simulink model "blockdiagram"  (R2020a)
settings: Solver=ode4  StartTime=0.0  StopTime=12  FixedStep=0.001  RelTol=1e-3
values from neighbouring files (symbols this model uses):
  B = 0.05    [ProblemA.m]
  J = 0.1    [ProblemA.m]
  L2 = (Lmax-Lmin)/2    (= 0.04)    [ProblemA.m]
  theta_m0 = 0    [ProblemA.m]
undefined symbols (not defined in the file or in its folder): sigbuilder_block
libraries: simulink x6
(part 1 of 2)
settings Model: Creator=IM SEYEONG  LastModifiedBy=IM SEYEONG

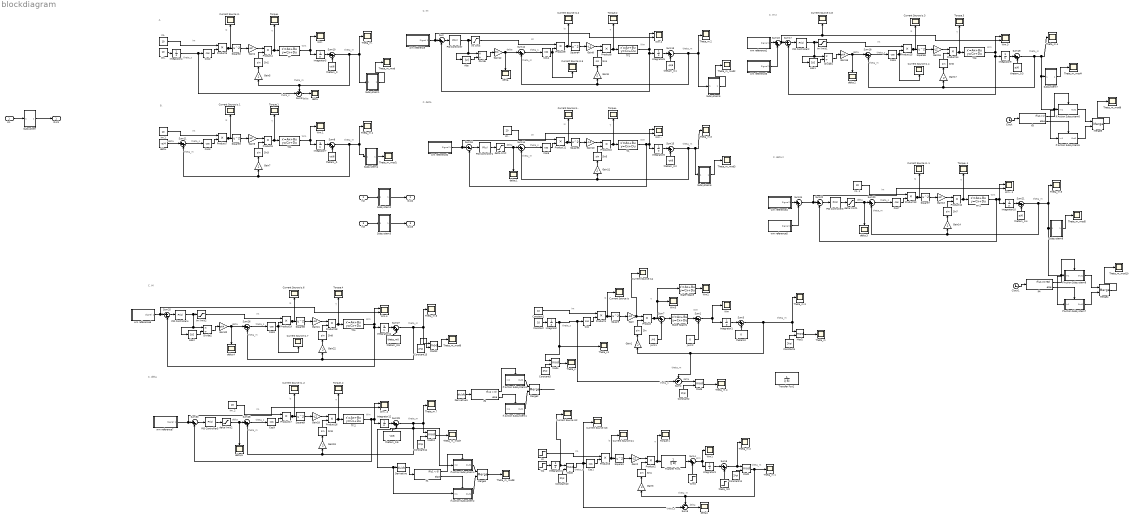
== system blockdiagram ==
  note: Wm
  note: T
  note: theta_m
  note: is
  note: theta_s
  note: Im
  note: theta_m
  note: theta_m
  note: Wm
  note: is
  note: theta_s
  note: delta
  note: T
  note: Im
  note: theta_s
  note: theta_m
  note: delta
  note: theta_s
  note: Wm
  note: theta_m
  note: theta_m
  note: is
  note: theta_s
  note: theta_s
  note: delta
  note: T
  note: Im
  note: A.
  note: B.
  note: T
  note: Im
  note: theta_m
  note: theta_s
  note: theta_m
  note: is
  note: Wm
  note: delta
  note: T
  note: theta_s
  note: theta_m
  note: Im
  note: C. IM
  note: is
  note: Wm
  note: delta
  note: theta_m
  note: T
  note: theta_s
  note: theta_m
  note: Im
  note: C. delta
  note: is
  note: Wm
  note: delta
  note: theta_m
  note: T
  note: C. delta 2
  note: delta
  note: Im
  note: theta_s
  note: theta_m
  note: theta_m
  note: Im
  note: C. IM 2
  note: is
  note: Wm
  note: Wm
  note: is
  note: T
  note: theta_s
  note: theta_m
  note: theta_m
  note: delta
  note: T
  note: C. delta
  note: delta
  note: Im
  note: theta_s
  note: theta_m
  note: theta_m
  note: Im
  note: C. IM
  note: is
  note: Wm
  note: Wm
  note: is
  note: T
  note: theta_s
  note: theta_m
  note: theta_m
  note: delta
  In1 : Inport
  In2 : Inport  Port=2
  In3 : Inport  Port=3
  Abs : Abs
  Abs1 : Abs
  Abs2 : Abs
  Clock : Clock
  Clock1 : Clock
  Constant : Constant  Value=10
  Constant1 : Constant  Value=10
  Constant{2,4..5,10..11,13..14} (7 alike) : Constant  Value=2*pi
  Cos{,1..9} (10 alike) : Trigonometry  Operator=cos
  Current Source is{,1..4} (5 alike) : Scope
  Current Source is.{,1..8} (9 alike) : Scope
  Current Source is.. : Scope
  Current Source is..1 : Scope
  Current Source is..2 : Scope
  Derivative : Derivative
  Derivative1 : Derivative
  Divide : Product  Inputs=*/
  Divide1 : Product  Inputs=*/
  Divide2 : Product  Inputs=*/
  Gain{,2,4,6,8,10,13,16,18,21} (10 alike) : Gain  Gain=-L2
  Gain{1,3,5,7,9,11,14,17,19,22} (10 alike) : Gain  Gain=2
  Gain12 : Gain  Gain=pi/4
  Gain15 : Gain  Gain=pi/4
  Gain20 : Gain  Gain=pi/4
  If Action Subsystem1 : Subsystem  TreatAsAtomicUnit=on
  If Action Subsystem2 : Subsystem  TreatAsAtomicUnit=on
  If Action Subsystem3 : Subsystem  TreatAsAtomicUnit=on
  If Action Subsystem4 : Subsystem  TreatAsAtomicUnit=on
  If Action Subsystem5 : Subsystem  TreatAsAtomicUnit=on
  If Action Subsystem6 : Subsystem  TreatAsAtomicUnit=on
  If Action Subsystem7 : Subsystem  TreatAsAtomicUnit=on
  If Action Subsystem8 : Subsystem  TreatAsAtomicUnit=on
  If1 : If  IfExpression=u1 < 0
  If2 : If  IfExpression=u1 < 0
  If3 : If  IfExpression=u1<1
  If4 : If  IfExpression=u1<0.732
  Im : Step  Time=0  After=10  SampleTime=0
  Im limit : Saturate  UpperLimit=20  LowerLimit=-20
  Im limit1 : Saturate  UpperLimit=20  LowerLimit=-20
  Im limit2 : Saturate  UpperLimit=20  LowerLimit=-20
  Im. : Constant  Value=10
  Im.. : Constant  Value=20
  Im..1 : Constant  Value=20
  Im..2 : Constant  Value=20
  Im.1 : Constant  Value=10
  Integrator{,1..12} (13 alike) : Integrator
  Jwm1 : Constant  Value=J*0
  Jwm2 : Constant  Value=0
  Merge{1..4} (4 alike) : Merge
  Mod{1..2,4..5,12..13} (6 alike) : Math  Operator=mod  SaturateOnIntegerOverflow=on
  Mod3 : Math  Operator=mod  OutputSignalType=real  SaturateOnIntegerOverflow=on
  PID Controller : simulink/Continuous/PID Controller  Controller=PI  Form=Parallel  TimeDomain=Continuous-time  UseExternalTs=off  SampleTime=-1  IntegratorMethod=Forward Euler  FilterMethod=Forward Euler  ControllerParametersSource=internal  P=4  I=0.9  D=0  UseFilter=on  N=100  TunerSelectOption=Transfer Function Based (PID Tuner App)  InitialConditionSource=internal  InitialConditionForIntegrator=0  InitialConditionForFilter=0  DifferentiatorICPrevScaledInput=0  ExternalReset=none  TrackingMode=off  Kt=1  LimitOutput=off  UpperSaturationLimit=inf  LowerSaturationLimit=-inf  LinearizeAsGain=on  AntiWindupMode=none  Kb=1  POutMin=[]  POutMax=[]  IOutMin=[]  IOutMax=[]  DOutMin=[]  DOutMax=[]  NOutMin=[]  NOutMax=[]  SumOutMin=[]  SumOutMax=[]  SaturationOutMin=[]  SaturationOutMax=[]  PParamMin=[]  PParamMax=[]  IParamMin=[]  IParamMax=[]  DParamMin=[]  DParamMax=[]  NParamMin=[]  NParamMax=[]  KbParamMin=[]  KbParamMax=[]  KtParamMin=[]  KtParamMax=[]  KbOutMin=[]  KbOutMax=[]  KtOutMin=[]  KtOutMax=[]  IntegratorOutMin=[]  IntegratorOutMax=[]  FilterOutMin=[]  FilterOutMax=[]  SumI1OutMin=[]  SumI1OutMax=[]  SumI2OutMin=[]  SumI2OutMax=[]  SumI3OutMin=[]  SumI3OutMax=[]  SumI4OutMin=[]  SumI4OutMax=[]  SumDOutMin=[]  SumDOutMax=[]  DifferentiatorOutMin=[]  DifferentiatorOutMax=[]  FilterDiffOutCoefMin=[]  FilterDiffOutCoefMax=[]  ReciprocalOutMin=[]  ReciprocalOutMax=[]  SumDenOutMin=[]  SumDenOutMax=[]  SumNumOutMin=[]  SumNumOutMax=[]  DivideOutMin=[]  DivideOutMax=[]  UdiffTsProdOutMin=[]  UdiffTsProdOutMax=[]  NTsProdOutMin=[]  NTsProdOutMax=[]  UintegralTsProdOutMin=[]  UintegralTsProdOutMax=[]  UngainTsProdOutMin=[]  UngainTsProdOutMax=[]  IntegratorContinuousStateAttributes=''  IntegratorStateMustResolveToSignalObject=off  IntegratorRTWStateStorageClass=Auto  FilterContinuousStateAttributes=''  FilterStateMustResolveToSignalObject=off  FilterRTWStateStorageClass=Auto  ParallelPVariant=InternalParameters  IdealPVariant=Disabled  IVariant=InternalParameters  DVariant=Disabled  IntegratorVariant=Continuous  SatVariant=Disabled  AWVariant=Passthrough  PCopyVariant=Disabled  TRVariant=Disabled  FdbkBlocksVariant=Forward  IdealPFdbkVariant=Disabled  SatFdbkVariant=Disabled  DerivativeFilterVariant=Disabled  NVariant=Disabled  NCopyVariant=Disabled_SignalSpec  FilterICVariant=Disabled  IntegratorICVariant=InternalICs  ExternalResetVariant=Disabled  TRSumVariant=Passthrough  SumFdbkVariant=Disabled  SumVariant=Sum_PI  TsampFilterVariant=InternalTs  TsampNgainVariant=Passthrough  TsampIntegralVariant=Passthrough
  PID Controller1 : simulink/Continuous/PID Controller  Controller=PI  Form=Parallel  TimeDomain=Continuous-time  UseExternalTs=off  SampleTime=-1  IntegratorMethod=Forward Euler  FilterMethod=Forward Euler  ControllerParametersSource=internal  P=1  I=0.05  D=0  UseFilter=on  N=100  TunerSelectOption=Transfer Function Based (PID Tuner App)  InitialConditionSource=internal  InitialConditionForIntegrator=0  InitialConditionForFilter=0  DifferentiatorICPrevScaledInput=0  ExternalReset=none  TrackingMode=off  Kt=1  LimitOutput=off  UpperSaturationLimit=inf  LowerSaturationLimit=-inf  LinearizeAsGain=on  AntiWindupMode=none  Kb=1  POutMin=[]  POutMax=[]  IOutMin=[]  IOutMax=[]  DOutMin=[]  DOutMax=[]  NOutMin=[]  NOutMax=[]  SumOutMin=[]  SumOutMax=[]  SaturationOutMin=[]  SaturationOutMax=[]  PParamMin=[]  PParamMax=[]  IParamMin=[]  IParamMax=[]  DParamMin=[]  DParamMax=[]  NParamMin=[]  NParamMax=[]  KbParamMin=[]  KbParamMax=[]  KtParamMin=[]  KtParamMax=[]  KbOutMin=[]  KbOutMax=[]  KtOutMin=[]  KtOutMax=[]  IntegratorOutMin=[]  IntegratorOutMax=[]  FilterOutMin=[]  FilterOutMax=[]  SumI1OutMin=[]  SumI1OutMax=[]  SumI2OutMin=[]  SumI2OutMax=[]  SumI3OutMin=[]  SumI3OutMax=[]  SumI4OutMin=[]  SumI4OutMax=[]  SumDOutMin=[]  SumDOutMax=[]  DifferentiatorOutMin=[]  DifferentiatorOutMax=[]  FilterDiffOutCoefMin=[]  FilterDiffOutCoefMax=[]  ReciprocalOutMin=[]  ReciprocalOutMax=[]  SumDenOutMin=[]  SumDenOutMax=[]  SumNumOutMin=[]  SumNumOutMax=[]  DivideOutMin=[]  DivideOutMax=[]  UdiffTsProdOutMin=[]  UdiffTsProdOutMax=[]  NTsProdOutMin=[]  NTsProdOutMax=[]  UintegralTsProdOutMin=[]  UintegralTsProdOutMax=[]  UngainTsProdOutMin=[]  UngainTsProdOutMax=[]  IntegratorContinuousStateAttributes=''  IntegratorStateMustResolveToSignalObject=off  IntegratorRTWStateStorageClass=Auto  FilterContinuousStateAttributes=''  FilterStateMustResolveToSignalObject=off  FilterRTWStateStorageClass=Auto  ParallelPVariant=InternalParameters  IdealPVariant=Disabled  IVariant=InternalParameters  DVariant=Disabled  IntegratorVariant=Continuous  SatVariant=Disabled  AWVariant=Passthrough  PCopyVariant=Disabled  TRVariant=Disabled  FdbkBlocksVariant=Forward  IdealPFdbkVariant=Disabled  SatFdbkVariant=Disabled  DerivativeFilterVariant=Disabled  NVariant=Disabled  NCopyVariant=Disabled_SignalSpec  FilterICVariant=Disabled  IntegratorICVariant=InternalICs  ExternalResetVariant=Disabled  TRSumVariant=Passthrough  SumFdbkVariant=Disabled  SumVariant=Sum_PI  TsampFilterVariant=InternalTs  TsampNgainVariant=Passthrough  TsampIntegralVariant=Passthrough
  PID Controller2 : simulink/Continuous/PID Controller  Controller=PI  Form=Parallel  TimeDomain=Continuous-time  UseExternalTs=off  SampleTime=-1  IntegratorMethod=Forward Euler  FilterMethod=Forward Euler  ControllerParametersSource=internal  P=4  I=0.9  D=0  UseFilter=on  N=100  TunerSelectOption=Transfer Function Based (PID Tuner App)  InitialConditionSource=internal  InitialConditionForIntegrator=0  InitialConditionForFilter=0  DifferentiatorICPrevScaledInput=0  ExternalReset=none  TrackingMode=off  Kt=1  LimitOutput=off  UpperSaturationLimit=inf  LowerSaturationLimit=-inf  LinearizeAsGain=on  AntiWindupMode=none  Kb=1  POutMin=[]  POutMax=[]  IOutMin=[]  IOutMax=[]  DOutMin=[]  DOutMax=[]  NOutMin=[]  NOutMax=[]  SumOutMin=[]  SumOutMax=[]  SaturationOutMin=[]  SaturationOutMax=[]  PParamMin=[]  PParamMax=[]  IParamMin=[]  IParamMax=[]  DParamMin=[]  DParamMax=[]  NParamMin=[]  NParamMax=[]  KbParamMin=[]  KbParamMax=[]  KtParamMin=[]  KtParamMax=[]  KbOutMin=[]  KbOutMax=[]  KtOutMin=[]  KtOutMax=[]  IntegratorOutMin=[]  IntegratorOutMax=[]  FilterOutMin=[]  FilterOutMax=[]  SumI1OutMin=[]  SumI1OutMax=[]  SumI2OutMin=[]  SumI2OutMax=[]  SumI3OutMin=[]  SumI3OutMax=[]  SumI4OutMin=[]  SumI4OutMax=[]  SumDOutMin=[]  SumDOutMax=[]  DifferentiatorOutMin=[]  DifferentiatorOutMax=[]  FilterDiffOutCoefMin=[]  FilterDiffOutCoefMax=[]  ReciprocalOutMin=[]  ReciprocalOutMax=[]  SumDenOutMin=[]  SumDenOutMax=[]  SumNumOutMin=[]  SumNumOutMax=[]  DivideOutMin=[]  DivideOutMax=[]  UdiffTsProdOutMin=[]  UdiffTsProdOutMax=[]  NTsProdOutMin=[]  NTsProdOutMax=[]  UintegralTsProdOutMin=[]  UintegralTsProdOutMax=[]  UngainTsProdOutMin=[]  UngainTsProdOutMax=[]  IntegratorContinuousStateAttributes=''  IntegratorStateMustResolveToSignalObject=off  IntegratorRTWStateStorageClass=Auto  FilterContinuousStateAttributes=''  FilterStateMustResolveToSignalObject=off  FilterRTWStateStorageClass=Auto  ParallelPVariant=InternalParameters  IdealPVariant=Disabled  IVariant=InternalParameters  DVariant=Disabled  IntegratorVariant=Continuous  SatVariant=Disabled  AWVariant=Passthrough  PCopyVariant=Disabled  TRVariant=Disabled  FdbkBlocksVariant=Forward  IdealPFdbkVariant=Disabled  SatFdbkVariant=Disabled  DerivativeFilterVariant=Disabled  NVariant=Disabled  NCopyVariant=Disabled_SignalSpec  FilterICVariant=Disabled  IntegratorICVariant=InternalICs  ExternalResetVariant=Disabled  TRSumVariant=Passthrough  SumFdbkVariant=Disabled  SumVariant=Sum_PI  TsampFilterVariant=InternalTs  TsampNgainVariant=Passthrough  TsampIntegralVariant=Passthrough
  PID Controller3 : simulink/Continuous/PID Controller  Controller=PI  Form=Parallel  TimeDomain=Continuous-time  UseExternalTs=off  SampleTime=-1  IntegratorMethod=Forward Euler  FilterMethod=Forward Euler  ControllerParametersSource=internal  P=1  I=0.05  D=0  UseFilter=on  N=100  TunerSelectOption=Transfer Function Based (PID Tuner App)  InitialConditionSource=internal  InitialConditionForIntegrator=0  InitialConditionForFilter=0  DifferentiatorICPrevScaledInput=0  ExternalReset=none  TrackingMode=off  Kt=1  LimitOutput=off  UpperSaturationLimit=inf  LowerSaturationLimit=-inf  LinearizeAsGain=on  AntiWindupMode=none  Kb=1  POutMin=[]  POutMax=[]  IOutMin=[]  IOutMax=[]  DOutMin=[]  DOutMax=[]  NOutMin=[]  NOutMax=[]  SumOutMin=[]  SumOutMax=[]  SaturationOutMin=[]  SaturationOutMax=[]  PParamMin=[]  PParamMax=[]  IParamMin=[]  IParamMax=[]  DParamMin=[]  DParamMax=[]  NParamMin=[]  NParamMax=[]  KbParamMin=[]  KbParamMax=[]  KtParamMin=[]  KtParamMax=[]  KbOutMin=[]  KbOutMax=[]  KtOutMin=[]  KtOutMax=[]  IntegratorOutMin=[]  IntegratorOutMax=[]  FilterOutMin=[]  FilterOutMax=[]  SumI1OutMin=[]  SumI1OutMax=[]  SumI2OutMin=[]  SumI2OutMax=[]  SumI3OutMin=[]  SumI3OutMax=[]  SumI4OutMin=[]  SumI4OutMax=[]  SumDOutMin=[]  SumDOutMax=[]  DifferentiatorOutMin=[]  DifferentiatorOutMax=[]  FilterDiffOutCoefMin=[]  FilterDiffOutCoefMax=[]  ReciprocalOutMin=[]  ReciprocalOutMax=[]  SumDenOutMin=[]  SumDenOutMax=[]  SumNumOutMin=[]  SumNumOutMax=[]  DivideOutMin=[]  DivideOutMax=[]  UdiffTsProdOutMin=[]  UdiffTsProdOutMax=[]  NTsProdOutMin=[]  NTsProdOutMax=[]  UintegralTsProdOutMin=[]  UintegralTsProdOutMax=[]  UngainTsProdOutMin=[]  UngainTsProdOutMax=[]  IntegratorContinuousStateAttributes=''  IntegratorStateMustResolveToSignalObject=off  IntegratorRTWStateStorageClass=Auto  FilterContinuousStateAttributes=''  FilterStateMustResolveToSignalObject=off  FilterRTWStateStorageClass=Auto  ParallelPVariant=InternalParameters  IdealPVariant=Disabled  IVariant=InternalParameters  DVariant=Disabled  IntegratorVariant=Continuous  SatVariant=Disabled  AWVariant=Passthrough  PCopyVariant=Disabled  TRVariant=Disabled  FdbkBlocksVariant=Forward  IdealPFdbkVariant=Disabled  SatFdbkVariant=Disabled  DerivativeFilterVariant=Disabled  NVariant=Disabled  NCopyVariant=Disabled_SignalSpec  FilterICVariant=Disabled  IntegratorICVariant=InternalICs  ExternalResetVariant=Disabled  TRSumVariant=Passthrough  SumFdbkVariant=Disabled  SumVariant=Sum_PI  TsampFilterVariant=InternalTs  TsampNgainVariant=Passthrough  TsampIntegralVariant=Passthrough
  PID Controller4 : simulink/Continuous/PID Controller  Controller=PI  Form=Parallel  TimeDomain=Continuous-time  UseExternalTs=off  SampleTime=-1  IntegratorMethod=Forward Euler  FilterMethod=Forward Euler  ControllerParametersSource=internal  P=4  I=0.9  D=0  UseFilter=on  N=100  TunerSelectOption=Transfer Function Based (PID Tuner App)  InitialConditionSource=internal  InitialConditionForIntegrator=0  InitialConditionForFilter=0  DifferentiatorICPrevScaledInput=0  ExternalReset=none  TrackingMode=off  Kt=1  LimitOutput=off  UpperSaturationLimit=inf  LowerSaturationLimit=-inf  LinearizeAsGain=on  AntiWindupMode=none  Kb=1  POutMin=[]  POutMax=[]  IOutMin=[]  IOutMax=[]  DOutMin=[]  DOutMax=[]  NOutMin=[]  NOutMax=[]  SumOutMin=[]  SumOutMax=[]  SaturationOutMin=[]  SaturationOutMax=[]  PParamMin=[]  PParamMax=[]  IParamMin=[]  IParamMax=[]  DParamMin=[]  DParamMax=[]  NParamMin=[]  NParamMax=[]  KbParamMin=[]  KbParamMax=[]  KtParamMin=[]  KtParamMax=[]  KbOutMin=[]  KbOutMax=[]  KtOutMin=[]  KtOutMax=[]  IntegratorOutMin=[]  IntegratorOutMax=[]  FilterOutMin=[]  FilterOutMax=[]  SumI1OutMin=[]  SumI1OutMax=[]  SumI2OutMin=[]  SumI2OutMax=[]  SumI3OutMin=[]  SumI3OutMax=[]  SumI4OutMin=[]  SumI4OutMax=[]  SumDOutMin=[]  SumDOutMax=[]  DifferentiatorOutMin=[]  DifferentiatorOutMax=[]  FilterDiffOutCoefMin=[]  FilterDiffOutCoefMax=[]  ReciprocalOutMin=[]  ReciprocalOutMax=[]  SumDenOutMin=[]  SumDenOutMax=[]  SumNumOutMin=[]  SumNumOutMax=[]  DivideOutMin=[]  DivideOutMax=[]  UdiffTsProdOutMin=[]  UdiffTsProdOutMax=[]  NTsProdOutMin=[]  NTsProdOutMax=[]  UintegralTsProdOutMin=[]  UintegralTsProdOutMax=[]  UngainTsProdOutMin=[]  UngainTsProdOutMax=[]  IntegratorContinuousStateAttributes=''  IntegratorStateMustResolveToSignalObject=off  IntegratorRTWStateStorageClass=Auto  FilterContinuousStateAttributes=''  FilterStateMustResolveToSignalObject=off  FilterRTWStateStorageClass=Auto  ParallelPVariant=InternalParameters  IdealPVariant=Disabled  IVariant=InternalParameters  DVariant=Disabled  IntegratorVariant=Continuous  SatVariant=Disabled  AWVariant=Passthrough  PCopyVariant=Disabled  TRVariant=Disabled  FdbkBlocksVariant=Forward  IdealPFdbkVariant=Disabled  SatFdbkVariant=Disabled  DerivativeFilterVariant=Disabled  NVariant=Disabled  NCopyVariant=Disabled_SignalSpec  FilterICVariant=Disabled  IntegratorICVariant=InternalICs  ExternalResetVariant=Disabled  TRSumVariant=Passthrough  SumFdbkVariant=Disabled  SumVariant=Sum_PI  TsampFilterVariant=InternalTs  TsampNgainVariant=Passthrough  TsampIntegralVariant=Passthrough
  PID Controller5 : simulink/Continuous/PID Controller  Controller=PI  Form=Parallel  TimeDomain=Continuous-time  UseExternalTs=off  SampleTime=-1  IntegratorMethod=Forward Euler  FilterMethod=Forward Euler  ControllerParametersSource=internal  P=1  I=0.05  D=0  UseFilter=on  N=100  TunerSelectOption=Transfer Function Based (PID Tuner App)  InitialConditionSource=internal  InitialConditionForIntegrator=0  InitialConditionForFilter=0  DifferentiatorICPrevScaledInput=0  ExternalReset=none  TrackingMode=off  Kt=1  LimitOutput=off  UpperSaturationLimit=inf  LowerSaturationLimit=-inf  LinearizeAsGain=on  AntiWindupMode=none  Kb=1  POutMin=[]  POutMax=[]  IOutMin=[]  IOutMax=[]  DOutMin=[]  DOutMax=[]  NOutMin=[]  NOutMax=[]  SumOutMin=[]  SumOutMax=[]  SaturationOutMin=[]  SaturationOutMax=[]  PParamMin=[]  PParamMax=[]  IParamMin=[]  IParamMax=[]  DParamMin=[]  DParamMax=[]  NParamMin=[]  NParamMax=[]  KbParamMin=[]  KbParamMax=[]  KtParamMin=[]  KtParamMax=[]  KbOutMin=[]  KbOutMax=[]  KtOutMin=[]  KtOutMax=[]  IntegratorOutMin=[]  IntegratorOutMax=[]  FilterOutMin=[]  FilterOutMax=[]  SumI1OutMin=[]  SumI1OutMax=[]  SumI2OutMin=[]  SumI2OutMax=[]  SumI3OutMin=[]  SumI3OutMax=[]  SumI4OutMin=[]  SumI4OutMax=[]  SumDOutMin=[]  SumDOutMax=[]  DifferentiatorOutMin=[]  DifferentiatorOutMax=[]  FilterDiffOutCoefMin=[]  FilterDiffOutCoefMax=[]  ReciprocalOutMin=[]  ReciprocalOutMax=[]  SumDenOutMin=[]  SumDenOutMax=[]  SumNumOutMin=[]  SumNumOutMax=[]  DivideOutMin=[]  DivideOutMax=[]  UdiffTsProdOutMin=[]  UdiffTsProdOutMax=[]  NTsProdOutMin=[]  NTsProdOutMax=[]  UintegralTsProdOutMin=[]  UintegralTsProdOutMax=[]  UngainTsProdOutMin=[]  UngainTsProdOutMax=[]  IntegratorContinuousStateAttributes=''  IntegratorStateMustResolveToSignalObject=off  IntegratorRTWStateStorageClass=Auto  FilterContinuousStateAttributes=''  FilterStateMustResolveToSignalObject=off  FilterRTWStateStorageClass=Auto  ParallelPVariant=InternalParameters  IdealPVariant=Disabled  IVariant=InternalParameters  DVariant=Disabled  IntegratorVariant=Continuous  SatVariant=Disabled  AWVariant=Passthrough  PCopyVariant=Disabled  TRVariant=Disabled  FdbkBlocksVariant=Forward  IdealPFdbkVariant=Disabled  SatFdbkVariant=Disabled  DerivativeFilterVariant=Disabled  NVariant=Disabled  NCopyVariant=Disabled_SignalSpec  FilterICVariant=Disabled  IntegratorICVariant=InternalICs  ExternalResetVariant=Disabled  TRSumVariant=Passthrough  SumFdbkVariant=Disabled  SumVariant=Sum_PI  TsampFilterVariant=InternalTs  TsampNgainVariant=Passthrough  TsampIntegralVariant=Passthrough
  Product{,1..19} (20 alike) : Product
  Sin{,1..9} (10 alike) : Trigonometry
  Square{,1..9} (10 alike) : Math  Operator=square  SaturateOnIntegerOverflow=on
  State-Space : StateSpace  A=-B/J  B=1/J  D=0  InitialCondition=10
  State-Space1 : StateSpace  A=-B/J  B=1/J  D=0  InitialCondition=10
  Subsystem : Subsystem
  Subsystem1 : Subsystem
  Subsystem2 : Subsystem
  Subsystem3 : Subsystem
  Subsystem4 : Subsystem
  Subsystem5 : Subsystem
  Subsystem6 : Subsystem
  Subsystem7 : Subsystem
  Subsystem8 : Subsystem
  Sum{,16..17,22,25,30} (6 alike) : Sum  Inputs=|+-
  Sum{1,3..4,6..8,10..15,18..21,23..24,26..29} (22 alike) : Sum  Inputs=|++
  Sum2 : Sum  Inputs=-+|
  Sum5 : Sum  Inputs=-+|
  Sum9 : Sum  Inputs=-+|
  TF : StateSpace  A=-B/J  B=1/J  D=0  InitialCondition=10
  TF, : StateSpace  A=-B/J  B=1/J  D=0  InitialCondition=0
  TF,1 : StateSpace  A=-B/J  B=1/J  D=0  InitialCondition=0
  TF,2 : StateSpace  A=-B/J  B=1/J  D=0  InitialCondition=0
  TF{1..4} (4 alike) : StateSpace  A=-B/J  B=1/J  D=0  InitialCondition=0
  Theta_m {,1..4} (5 alike) : Scope
  Theta_m.{,1..7} (8 alike) : Scope
  Theta_m_mod{,1..10} (11 alike) : Scope
  Theta_s : Scope
  Theta_s1 : Scope
  Torque 1 : Scope
  Torque.{,1..4} (5 alike) : Scope
  Torque.. : Scope
  Torque..1 : Scope
  Torque..2 : Scope
  Transfer Fcn1 : TransferFcn  Denominator=[J B]
  Transfer Fcn2 : TransferFcn  Denominator=[J B]
  Wm{,1..3} (4 alike) : Scope
  Wm. : Scope
  Wm... : Scope  NumInputPorts=2
  Wm...1 : Scope  NumInputPorts=2
  Wm...2 : Scope  NumInputPorts=2
  Wm.1 : Scope
  Wm.2 : Scope  NumInputPorts=2
  Wm.3 : Scope  NumInputPorts=2
  Wm.4 : Scope  NumInputPorts=2
  Wm0 : Step  Time=0  After=0  SampleTime=0
  Ws : Step  Time=0  After=10  SampleTime=0
  Ws. : Constant  Value=10
  delta : Scope
  delta limit : Saturate  UpperLimit=pi/4  LowerLimit=-pi/4
  delta limit1 : Saturate  UpperLimit=pi/4  LowerLimit=-pi/4
  delta limit2 : Saturate  UpperLimit=pi/4  LowerLimit=-pi/4
  delta,{,1..5} (6 alike) : Scope
  delta. : Constant  Value=-pi/4
  delta1 : Scope
  theta_m0 : Step  Time=0  After=pi/6  SampleTime=0
  thetam0 : Constant  Value=0
  thetam_0 : Constant  Value=-pi/6
  thetam_0.{,1..2,6} (4 alike) : Constant  Value=-pi/6
  thetam_0.3 : Constant  Value=pi/6
  thetam_0.4 : Constant  Value=pi/6
  thetam_0.5 : Constant  Value=theta_m0
  wm reference : Subsystem  Tag=STV Subsys  LoadFcn=sigbuilder_block('load');  StartFcn=sigbuilder_block('start');  StopFcn=sigbuilder_block('stop');  ClipboardFcn=sigbuilder_block('clipboard');  mask(Sigbuilder block){tuvar=[0:10]}
      mask help: Simulink:masks:SigbuilderBlock_MD
      mask init:
      | if ~strcmp(get_param(bdroot(gcbh),'SimulationStatus'),'stopped') tuvar = sigbuilder_block('maskInit'); end
      settings: CopyFcn=sigbuilder_block('copy');  DeleteFcn=sigbuilder_block('delete');  ModelCloseFcn=sigbuilder_block('modelClose');  PreSaveFcn=sigbuilder_block('preSave');  PauseFcn=sigbuilder_block('pause');  ContinueFcn=sigbuilder_block('continue');  NameChangeFcn=sigbuilder_block('namechange');  OpenFcn=sigbuilder_block('open',[433.5 195.75 558 399.75 ]);  CloseFcn=sigbuilder_block('close');
      mask Display: plot(0, 0, 100, 100,[2, 2, 32, 32, 2], [68, 8, 8, 68, 68],[32, 2], [38, 38], [32, 19, 2],[53, 60, 44], [32, 17, 17, 2],[16, 16, 31, 31]);txt = getActiveGroup(gcbh);text(2, 100, txt,'verticalAlignment', 'top');
  wm reference1 : Subsystem  Tag=STV Subsys  LoadFcn=sigbuilder_block('load');  StartFcn=sigbuilder_block('start');  StopFcn=sigbuilder_block('stop');  ClipboardFcn=sigbuilder_block('clipboard');  mask(Sigbuilder block){tuvar=[0:10]}
      mask help: Simulink:masks:SigbuilderBlock_MD
      mask init:
      | if ~strcmp(get_param(bdroot(gcbh),'SimulationStatus'),'stopped') tuvar = sigbuilder_block('maskInit'); end
      settings: CopyFcn=sigbuilder_block('copy');  DeleteFcn=sigbuilder_block('delete');  ModelCloseFcn=sigbuilder_block('modelClose');  PreSaveFcn=sigbuilder_block('preSave');  PauseFcn=sigbuilder_block('pause');  ContinueFcn=sigbuilder_block('continue');  NameChangeFcn=sigbuilder_block('namechange');  OpenFcn=sigbuilder_block('open',[408.6 126 558 400.2 ]);  CloseFcn=sigbuilder_block('close');
      mask Display: plot(0, 0, 100, 100,[2, 2, 32, 32, 2], [68, 8, 8, 68, 68],[32, 2], [38, 38], [32, 19, 2],[53, 60, 44], [32, 17, 17, 2],[16, 16, 31, 31]);txt = getActiveGroup(gcbh);text(2, 100, txt,'verticalAlignment', 'top');
  wm reference2 : Subsystem  Tag=STV Subsys  LoadFcn=sigbuilder_block('load');  StartFcn=sigbuilder_block('start');  StopFcn=sigbuilder_block('stop');  ClipboardFcn=sigbuilder_block('clipboard');  mask(Sigbuilder block){tuvar=[0:10]}
      mask help: Simulink:masks:SigbuilderBlock_MD
      mask init:
      | if ~strcmp(get_param(bdroot(gcbh),'SimulationStatus'),'stopped') tuvar = sigbuilder_block('maskInit'); end
      settings: CopyFcn=sigbuilder_block('copy');  DeleteFcn=sigbuilder_block('delete');  ModelCloseFcn=sigbuilder_block('modelClose');  PreSaveFcn=sigbuilder_block('preSave');  PauseFcn=sigbuilder_block('pause');  ContinueFcn=sigbuilder_block('continue');  NameChangeFcn=sigbuilder_block('namechange');  OpenFcn=sigbuilder_block('open',[433.5 195.75 558 399.75 ]);  CloseFcn=sigbuilder_block('close');
      mask Display: plot(0, 0, 100, 100,[2, 2, 32, 32, 2], [68, 8, 8, 68, 68],[32, 2], [38, 38], [32, 19, 2],[53, 60, 44], [32, 17, 17, 2],[16, 16, 31, 31]);txt = getActiveGroup(gcbh);text(2, 100, txt,'verticalAlignment', 'top');
  wm reference3 : Subsystem  Tag=STV Subsys  LoadFcn=sigbuilder_block('load');  StartFcn=sigbuilder_block('start');  StopFcn=sigbuilder_block('stop');  ClipboardFcn=sigbuilder_block('clipboard');  mask(Sigbuilder block){tuvar=[0:10]}
      mask help: Simulink:masks:SigbuilderBlock_MD
      mask init:
      | if ~strcmp(get_param(bdroot(gcbh),'SimulationStatus'),'stopped') tuvar = sigbuilder_block('maskInit'); end
      settings: CopyFcn=sigbuilder_block('copy');  DeleteFcn=sigbuilder_block('delete');  ModelCloseFcn=sigbuilder_block('modelClose');  PreSaveFcn=sigbuilder_block('preSave');  PauseFcn=sigbuilder_block('pause');  ContinueFcn=sigbuilder_block('continue');  NameChangeFcn=sigbuilder_block('namechange');  OpenFcn=sigbuilder_block('open',[361.2 123.6 558 400.2 ]);  CloseFcn=sigbuilder_block('close');
      mask Display: plot(0, 0, 100, 100,[2, 2, 32, 32, 2], [68, 8, 8, 68, 68],[32, 2], [38, 38], [32, 19, 2],[53, 60, 44], [32, 17, 17, 2],[16, 16, 31, 31]);txt = getActiveGroup(gcbh);text(2, 100, txt,'verticalAlignment', 'top');
  wm reference4 : Subsystem  Tag=STV Subsys  LoadFcn=sigbuilder_block('load');  StartFcn=sigbuilder_block('start');  StopFcn=sigbuilder_block('stop');  ClipboardFcn=sigbuilder_block('clipboard');  mask(Sigbuilder block){tuvar=[0:10]}
      mask help: Simulink:masks:SigbuilderBlock_MD
      mask init:
      | if ~strcmp(get_param(bdroot(gcbh),'SimulationStatus'),'stopped') tuvar = sigbuilder_block('maskInit'); end
      settings: CopyFcn=sigbuilder_block('copy');  DeleteFcn=sigbuilder_block('delete');  ModelCloseFcn=sigbuilder_block('modelClose');  PreSaveFcn=sigbuilder_block('preSave');  PauseFcn=sigbuilder_block('pause');  ContinueFcn=sigbuilder_block('continue');  NameChangeFcn=sigbuilder_block('namechange');  OpenFcn=sigbuilder_block('open',[408.6 126 558 400.2 ]);  CloseFcn=sigbuilder_block('close');
      mask Display: plot(0, 0, 100, 100,[2, 2, 32, 32, 2], [68, 8, 8, 68, 68],[32, 2], [38, 38], [32, 19, 2],[53, 60, 44], [32, 17, 17, 2],[16, 16, 31, 31]);txt = getActiveGroup(gcbh);text(2, 100, txt,'verticalAlignment', 'top');
  wm reference5 : Subsystem  Tag=STV Subsys  LoadFcn=sigbuilder_block('load');  StartFcn=sigbuilder_block('start');  StopFcn=sigbuilder_block('stop');  ClipboardFcn=sigbuilder_block('clipboard');  mask(Sigbuilder block){tuvar=[0:10]}
      mask help: Simulink:masks:SigbuilderBlock_MD
      mask init:
      | if ~strcmp(get_param(bdroot(gcbh),'SimulationStatus'),'stopped') tuvar = sigbuilder_block('maskInit'); end
      settings: CopyFcn=sigbuilder_block('copy');  DeleteFcn=sigbuilder_block('delete');  ModelCloseFcn=sigbuilder_block('modelClose');  PreSaveFcn=sigbuilder_block('preSave');  PauseFcn=sigbuilder_block('pause');  ContinueFcn=sigbuilder_block('continue');  NameChangeFcn=sigbuilder_block('namechange');  OpenFcn=sigbuilder_block('open',[361.2 123.6 558 400.2 ]);  CloseFcn=sigbuilder_block('close');
      mask Display: plot(0, 0, 100, 100,[2, 2, 32, 32, 2], [68, 8, 8, 68, 68],[32, 2], [38, 38], [32, 19, 2],[53, 60, 44], [32, 17, 17, 2],[16, 16, 31, 31]);txt = getActiveGroup(gcbh);text(2, 100, txt,'verticalAlignment', 'top');
  wm reference6 : Subsystem  Tag=STV Subsys  LoadFcn=sigbuilder_block('load');  StartFcn=sigbuilder_block('start');  StopFcn=sigbuilder_block('stop');  ClipboardFcn=sigbuilder_block('clipboard');  mask(Sigbuilder block){tuvar=[0:10]}
      mask help: Simulink:masks:SigbuilderBlock_MD
      mask init:
      | if ~strcmp(get_param(bdroot(gcbh),'SimulationStatus'),'stopped') tuvar = sigbuilder_block('maskInit'); end
      settings: CopyFcn=sigbuilder_block('copy');  DeleteFcn=sigbuilder_block('delete');  ModelCloseFcn=sigbuilder_block('modelClose');  PreSaveFcn=sigbuilder_block('preSave');  PauseFcn=sigbuilder_block('pause');  ContinueFcn=sigbuilder_block('continue');  NameChangeFcn=sigbuilder_block('namechange');  OpenFcn=sigbuilder_block('open',[433.5 195.75 558 399.75 ]);  CloseFcn=sigbuilder_block('close');
      mask Display: plot(0, 0, 100, 100,[2, 2, 32, 32, 2], [68, 8, 8, 68, 68],[32, 2], [38, 38], [32, 19, 2],[53, 60, 44], [32, 17, 17, 2],[16, 16, 31, 31]);txt = getActiveGroup(gcbh);text(2, 100, txt,'verticalAlignment', 'top');
  wm reference7 : Subsystem  Tag=STV Subsys  LoadFcn=sigbuilder_block('load');  StartFcn=sigbuilder_block('start');  StopFcn=sigbuilder_block('stop');  ClipboardFcn=sigbuilder_block('clipboard');  mask(Sigbuilder block){tuvar=[0:10]}
      mask help: Simulink:masks:SigbuilderBlock_MD
      mask init:
      | if ~strcmp(get_param(bdroot(gcbh),'SimulationStatus'),'stopped') tuvar = sigbuilder_block('maskInit'); end
      settings: CopyFcn=sigbuilder_block('copy');  DeleteFcn=sigbuilder_block('delete');  ModelCloseFcn=sigbuilder_block('modelClose');  PreSaveFcn=sigbuilder_block('preSave');  PauseFcn=sigbuilder_block('pause');  ContinueFcn=sigbuilder_block('continue');  NameChangeFcn=sigbuilder_block('namechange');  OpenFcn=sigbuilder_block('open',[433.5 195.75 558 399.75 ]);  CloseFcn=sigbuilder_block('close');
      mask Display: plot(0, 0, 100, 100,[2, 2, 32, 32, 2], [68, 8, 8, 68, 68],[32, 2], [38, 38], [32, 19, 2],[53, 60, 44], [32, 17, 17, 2],[16, 16, 31, 31]);txt = getActiveGroup(gcbh);text(2, 100, txt,'verticalAlignment', 'top');
  Out1 : Outport
  Out2 : Outport  Port=2
  Out3 : Outport  Port=3
  wires:
  Constant/1 -> Integrator/1
  Constant1/1 -> Product1/1
  Cos/1 -> Product1/2
  Product1/1 -> Current Source is/1, Square/1
  Square/1 -> Gain/1
  Gain/1 -> Current Source is4/1, Product/1
  Gain1/1 -> Sin/1
  Sin/1 -> Product/2
  theta_m0/1 -> Sum6/2
  Gain2/1 -> Product2/1
  Constant11/1 -> Mod2/2
  Sin1/1 -> Product2/2
  Im/1 -> Product3/1
  Square1/1 -> Gain2/1
  Mod2/1 -> Gain3/1, Sum5/1, Theta_m 1/1
  Constant10/1 -> Mod3/2
  Product3/1 -> Current Source is1/1, Square1/1
  Mod3/1 -> Sum5/2, Cos1/1, Current Source is3/1
  Integrator3/1 -> Sum6/1
  Product2/1 -> Torque 1/1, Transfer Fcn1/1
  Integrator2/1 -> Current Source is2/1, Mod3/1
  Transfer Fcn1/1 -> Sum4/1
  Gain3/1 -> Sin1/1
  Sum5/1 -> delta1/1
  Sum6/1 -> Theta_m 2/1, Mod2/1
  Sum4/1 -> Integrator3/1, Wm1/1
  Cos1/1 -> Product3/2
  Ws/1 -> Integrator2/1
  Wm0/1 -> Sum4/2
  Constant4/1 -> Mod1/2
  Mod1/1 -> "Theta_m "/1
  Integrator/1 -> Theta_s1/1, Mod4/1, Sum2/2, Cos/1
  Sum3/1 -> Gain1/1, Sum2/1, Mod1/1, Theta_m 3/1
  Sum2/1 -> Mod5/1
  Constant5/1 -> Mod4/2
  Mod4/1 -> Theta_s/1
  Constant2/1 -> Mod5/2
  Mod5/1 -> Theta_m 4/1
  Jwm1/1 -> Sum7/2
  Jwm2/1 -> Sum1/2
  Sum1/1 -> Integrator1/1, Wm/1
  thetam0/1 -> Sum3/2
  Integrator1/1 -> Sum3/1
  Product/1 -> Wm3/1, State-Space/1, Sum7/1
  State-Space/1 -> Wm2/1
  State-Space1/1 -> Sum1/1
  Sum7/1 -> State-Space1/1
  Integrator5/1 -> Sum10/1
  thetam_0/1 -> Sum10/2
  Integrator4/1 -> Sum9/2, Cos2/1
  Sum10/1 -> Gain5/1, Sum9/1, Subsystem1/1(In1), Theta_m./1
  Ws./1 -> Integrator4/1
  TF/1 -> Integrator5/1, Wm./1
  Square2/1 -> Gain4/1
  Gain4/1 -> Product4/1
  Sin2/1 -> Product4/2
  Gain5/1 -> Sin2/1
  Product5/1 -> Current Source is./1, Square2/1
  Im./1 -> Product5/1
  Cos2/1 -> Product5/2
  Product4/1 -> TF/1, Torque./1
  Sum9/1 -> delta/1
  Product6/1 -> TF1/1, Torque.1/1
  Cos3/1 -> Product7/2
  Product7/1 -> Current Source is.1/1, Square3/1
  Gain7/1 -> Sin3/1
  Sin3/1 -> Product6/2
  Gain6/1 -> Product6/1
  TF1/1 -> Integrator7/1, Wm.1/1
  delta./1 -> Sum11/1
  Im.1/1 -> Product7/1
  thetam_0./1 -> Sum8/2
  Sum8/1 -> Gain7/1, Sum11/2, Subsystem4/1(In1), Theta_m.1/1
  Integrator7/1 -> Sum8/1
  Square3/1 -> Gain6/1
  Sum11/1 -> Cos3/1
  Sum12/1 -> Cos4/1
  Square4/1 -> Gain8/1
  Cos4/1 -> Current Source is.5/1, Product9/2
  thetam_0.1/1 -> Sum13/2
  Gain9/1 -> Sin4/1
  Sum13/1 -> Gain9/1, Sum12/2, Subsystem5/1(In1), Theta_m.2/1
  Subsystem5/1(Out1) -> Theta_m_mod2/1
  Im limit/1 -> Product9/1
  Integrator6/1 -> Sum13/1
  TF2/1 -> Sum/2, Integrator6/1, Wm.2/1
  Gain8/1 -> Product8/1
  Product9/1 -> Current Source is.2/1, Square4/1
  Sin4/1 -> Product8/2
  Product8/1 -> TF2/1, Torque.2/1
  Sum14/1 -> Cos5/1
  Square5/1 -> Gain10/1
  Cos5/1 -> Product11/2
  thetam_0.2/1 -> Sum15/2
  Gain11/1 -> Sin5/1
  Sum15/1 -> Gain11/1, Sum14/2, Subsystem6/1(In1), Theta_m.3/1
  Subsystem6/1(Out1) -> Theta_m_mod3/1
  Im../1 -> Product11/1
  Integrator8/1 -> Sum15/1
  TF,/1 -> Wm.../1, Integrator8/1, Sum16/2
  Gain10/1 -> Product10/1
  delta limit/1 -> Sum14/1, delta,1/1
  Product11/1 -> Current Source is../1, Square5/1
  Sin5/1 -> Product10/2
  Product10/1 -> TF,/1, Torque../1
  Sum/1 -> PID Controller/1
  wm reference/1(Signal 1) -> Wm.2/2, Sum/1
  PID Controller/1 -> Abs/1, Divide/1, Im limit/1
  Gain12/1 -> delta,/1, Sum12/1
  Divide/1 -> Gain12/1
  Abs/1 -> Divide/2
  Sum16/1 -> PID Controller1/1
  wm reference2/1(Signal 1) -> Wm.../2, Sum16/1
  PID Controller1/1 -> delta limit/1
  Sum24/1 -> Wm...1/2, Sum22/1
  PID Controller3/1 -> delta limit1/1
  Product14/1 -> TF3/1, Torque.3/1
  Square7/1 -> Gain13/1
  Sum22/1 -> PID Controller3/1
  Gain15/1 -> delta,2/1, Sum18/1
  PID Controller2/1 -> Abs1/1, Divide1/1, Im limit1/1
  Abs1/1 -> Divide1/2
  TF3/1 -> Sum17/2, Integrator9/1, Wm.3/1
  Sin7/1 -> Product12/2
  Sum17/1 -> PID Controller2/1
  Gain13/1 -> Product12/1
  delta limit1/1 -> Sum20/1, delta,3/1
  Gain16/1 -> Product14/1
  Subsystem8/1(Out1) -> Theta_m_mod5/1
  Im..1/1 -> Product13/1
  Integrator10/1 -> Sum21/1
  Gain14/1 -> Sin7/1
  Cos7/1 -> Product13/2
  thetam_0.4/1 -> Sum21/2
  Im limit1/1 -> Product15/1
  Sin6/1 -> Product14/2
  Integrator9/1 -> Sum19/1
  Product15/1 -> Current Source is.3/1, Square6/1
  Sum18/1 -> Cos6/1
  Gain17/1 -> Sin6/1
  Square6/1 -> Gain16/1
  Subsystem7/1(Out1) -> Theta_m_mod4/1
  Product12/1 -> TF,1/1, Torque..1/1
  Cos6/1 -> Current Source is.4/1, Product15/2
  Product13/1 -> Current Source is..1/1, Square7/1
  Sum19/1 -> Gain17/1, Sum18/2, If Action Subsystem5/1(In1), If Action Subsystem6/1(In1), Subsystem7/1(In1), Theta_m.4/1
  Sum20/1 -> Cos7/1
  TF,1/1 -> Wm...1/1, Integrator10/1, Sum22/2
  Divide1/1 -> Gain15/1
  thetam_0.3/1 -> Sum19/2
  wm reference1/1(Signal 1) -> Sum23/1
  Sum23/1 -> Current Source is.8/1, Wm.3/2, Sum17/1
  wm reference3/1(Signal 1) -> Sum23/2
  wm reference5/1(Signal 1) -> Sum24/2
  wm reference4/1(Signal 1) -> Sum24/1
  PID Controller5/1 -> delta limit2/1
  Product18/1 -> TF4/1, Torque.4/1
  Square9/1 -> Gain18/1
  Sum30/1 -> PID Controller5/1
  Gain20/1 -> delta,4/1, Sum26/1
  PID Controller4/1 -> Abs2/1, Divide2/1, Im limit2/1
  wm reference7/1(Signal 1) -> Wm...2/2, Sum30/1
  Abs2/1 -> Divide2/2
  TF4/1 -> Sum25/2, Integrator11/1, Wm.4/1
  Constant13/1 -> Mod12/2
  Sin9/1 -> Product16/2
  Sum25/1 -> PID Controller4/1
  Gain18/1 -> Product16/1
  Constant14/1 -> Mod13/2
  delta limit2/1 -> Sum28/1, delta,5/1
  Gain21/1 -> Product18/1
  Mod13/1 -> Theta_m_mod7/1
  Im..2/1 -> Product17/1
  Integrator12/1 -> Sum29/1
  Sum29/1 -> If Action Subsystem4/1(In2), If Action Subsystem2/1(In1), Derivative/1, Gain19/1, Sum28/2, Mod13/1, Theta_m.7/1
  Gain19/1 -> Sin9/1
  Cos9/1 -> Product17/2
  thetam_0.6/1 -> Sum29/2
  Im limit2/1 -> Product19/1
  Sin8/1 -> Product18/2
  Integrator11/1 -> Sum27/1
  Product19/1 -> Current Source is.6/1, Square8/1
  Sum26/1 -> Cos8/1
  Gain22/1 -> Sin8/1
  Square8/1 -> Gain21/1
  Mod12/1 -> Theta_m_mod6/1
  Product16/1 -> TF,2/1, Torque..2/1
  wm reference6/1(Signal 1) -> Wm.4/2, Sum25/1
  Cos8/1 -> Current Source is.7/1, Product19/2
  Product17/1 -> Current Source is..2/1, Square9/1
  Sum27/1 -> Gain22/1, Sum26/2, Mod12/1, Theta_m.6/1
  Sum28/1 -> Cos9/1
  TF,2/1 -> Wm...2/1, Integrator12/1, Sum30/2
  Divide2/1 -> Gain20/1
  thetam_0.5/1 -> Sum27/2
  Merge1/1 -> Theta_m_mod8/1
  If Action Subsystem2/1(Out1) -> Merge1/2
  If1/2 -> If Action Subsystem2/Action
  If1/1 -> If Action Subsystem4/Action
  Derivative/1 -> If1/1
  In1/1 -> Subsystem/1(In1)
  Subsystem/1(Out1) -> Out1/1
  Subsystem1/1(Out1) -> Theta_m_mod/1
  Subsystem2/1(Out1) -> Out2/1
  In2/1 -> Subsystem2/1(In1)
  Subsystem3/1(Out1) -> Out3/1
  In3/1 -> Subsystem3/1(In1)
  If Action Subsystem4/1(Out2) -> Merge1/1
  Subsystem4/1(Out1) -> Theta_m_mod1/1
  If Action Subsystem3/1(Out2) -> Merge2/1
  If2/1 -> If Action Subsystem3/Action
  If2/2 -> If Action Subsystem1/Action
  Merge2/1 -> ?
  If Action Subsystem1/1(Out1) -> Merge2/2
  Derivative1/1 -> If2/1
  ? -> Derivative1/1
  Clock/1 -> If3/1
  If3/1 -> If Action Subsystem6/Action
  If3/2 -> If Action Subsystem5/Action
  If Action Subsystem6/1(Out1) -> Merge3/1
  If Action Subsystem5/1(Out1) -> Merge3/2
  Merge3/1 -> Theta_m_mod9/1
  If Action Subsystem7/1(Out1) -> Merge4/2
  Clock1/1 -> If4/1
  Sum21/1 -> Gain14/1, Sum20/2, If Action Subsystem7/1(In1), If Action Subsystem8/1(In1), Subsystem8/1(In1), Theta_m.5/1
  If Action Subsystem8/1(Out1) -> Merge4/1
  Merge4/1 -> Theta_m_mod10/1
  If4/1 -> If Action Subsystem8/Action
  If4/2 -> If Action Subsystem7/Action

== system blockdiagram/If Action Subsystem1 ==
  In1 : Inport
  Action Port : ActionPort  ActionPortLabel=else
  If Action Subsystem2 : Subsystem  TreatAsAtomicUnit=on
  If Action Subsystem4 : Subsystem  TreatAsAtomicUnit=on
  If1 : If  IfExpression=u1 <ep
  Merge1 : Merge
  Out1 : Outport
  wires:
  If1/1 -> If Action Subsystem4/Action
  If1/2 -> If Action Subsystem2/Action
  Merge1/1 -> Out1/1
  If Action Subsystem4/1(Out1) -> Merge1/1
  If Action Subsystem2/1(Out1) -> Merge1/2
  In1/1 -> If Action Subsystem2/1(In1), If Action Subsystem4/1(In1), If1/1

== system blockdiagram/If Action Subsystem2 ==
  In1 : Inport
  Action Port : ActionPort  ActionPortLabel=else
  If Action Subsystem2 : Subsystem  TreatAsAtomicUnit=on
  If Action Subsystem4 : Subsystem  TreatAsAtomicUnit=on
  If1 : If  IfExpression=u1 <ep
  Merge1 : Merge
  Out1 : Outport
  wires:
  If1/1 -> If Action Subsystem4/Action
  If1/2 -> If Action Subsystem2/Action
  Merge1/1 -> Out1/1
  If Action Subsystem4/1(Out1) -> Merge1/1
  If Action Subsystem2/1(Out1) -> Merge1/2
  In1/1 -> If Action Subsystem2/1(In1), If Action Subsystem4/1(In1), If1/1

== system blockdiagram/If Action Subsystem3 ==
  In2 : Inport
  Action Port : ActionPort  InitializeStates=reset  ActionPortLabel=if(u1 < 0)
  Add : Sum  Inputs=+-
  Constant : Constant  Value=2*pi
  Constant14 : Constant  Value=-2*pi
  If Action Subsystem1 : Subsystem  TreatAsAtomicUnit=on
  If Action Subsystem3 : Subsystem  TreatAsAtomicUnit=on
  If2 : If  IfExpression=u1 <-ep
  Merge2 : Merge
  Mod13 : Math  Operator=mod  SaturateOnIntegerOverflow=on
  Out2 : Outport
  wires:
  Mod13/1 -> ?
  Constant14/1 -> Mod13/2
  ? -> Mod13/1
  Constant/1 -> Add/2
  In2/1 -> If Action Subsystem1/1(In1), If Action Subsystem3/1(In1), If2/1
  If Action Subsystem3/1(Out1) -> Merge2/1
  If2/1 -> If Action Subsystem3/Action
  If Action Subsystem1/1(Out1) -> Merge2/2
  If2/2 -> If Action Subsystem1/Action
  Merge2/1 -> Out2/1

== system blockdiagram/If Action Subsystem4 ==
  In2 : Inport
  Action Port : ActionPort  InitializeStates=reset  ActionPortLabel=if(u1 < 0)
  Add : Sum  Inputs=+-
  Constant : Constant  Value=2*pi
  Constant14 : Constant  Value=-2*pi
  If Action Subsystem1 : Subsystem  TreatAsAtomicUnit=on
  If Action Subsystem3 : Subsystem  TreatAsAtomicUnit=on
  If2 : If  IfExpression=u1 <-ep
  Merge2 : Merge
  Mod13 : Math  Operator=mod  SaturateOnIntegerOverflow=on
  Out2 : Outport
  wires:
  Mod13/1 -> ?
  Constant14/1 -> Mod13/2
  ? -> Mod13/1
  Constant/1 -> Add/2
  In2/1 -> If Action Subsystem1/1(In1), If Action Subsystem3/1(In1), If2/1
  If Action Subsystem3/1(Out1) -> Merge2/1
  If2/1 -> If Action Subsystem3/Action
  If Action Subsystem1/1(Out1) -> Merge2/2
  If2/2 -> If Action Subsystem1/Action
  Merge2/1 -> Out2/1

== system blockdiagram/If Action Subsystem5 ==
  In1 : Inport
  Action Port : ActionPort  ActionPortLabel=else
  Subsystem7 : Subsystem
  Out1 : Outport
  wires:
  In1/1 -> Subsystem7/1(In1)
  Subsystem7/1(Out1) -> Out1/1

== system blockdiagram/If Action Subsystem6 ==
  In1 : Inport
  Action Port : ActionPort  InitializeStates=reset  ActionPortLabel=if(u1<1)
  Out1 : Outport
  wires:
  In1/1 -> Out1/1

== system blockdiagram/If Action Subsystem7 ==
  In1 : Inport
  Action Port : ActionPort  ActionPortLabel=else
  Clock1 : Clock
  If Action Subsystem1 : Subsystem  TreatAsAtomicUnit=on
  If Action Subsystem7 : Subsystem  TreatAsAtomicUnit=on
  If4 : If  IfExpression=u1<1.772
  Merge2 : Merge
  Subsystem7 : Subsystem
  Out1 : Outport
  wires:
  Merge2/1 -> Out1/1
  If4/1 -> If Action Subsystem1/Action
  If4/2 -> If Action Subsystem7/Action
  In1/1 -> If Action Subsystem1/1(In1), If Action Subsystem7/1(In1)
  Clock1/1 -> If4/1
  If Action Subsystem1/1(Out1) -> Merge2/1
  If Action Subsystem7/1(Out1) -> Merge2/2

== system blockdiagram/If Action Subsystem8 ==
  In1 : Inport
  Action Port : ActionPort  InitializeStates=reset  ActionPortLabel=if(u1<0.732)
  Out1 : Outport
  wires:
  In1/1 -> Out1/1

== system blockdiagram/Subsystem ==
  In1 : Inport
  Derivative1 : Derivative
  If Action Subsystem1 : Subsystem  TreatAsAtomicUnit=on
  If Action Subsystem3 : Subsystem  TreatAsAtomicUnit=on
  If2 : If  IfExpression=u1 < 0
  Merge2 : Merge
  Out1 : Outport
  wires:
  Derivative1/1 -> If2/1
  If2/2 -> If Action Subsystem1/Action
  If Action Subsystem1/1(Out1) -> Merge2/2
  If Action Subsystem3/1(Out2) -> Merge2/1
  If2/1 -> If Action Subsystem3/Action
  In1/1 -> If Action Subsystem3/1(In2), If Action Subsystem1/1(In1), Derivative1/1
  Merge2/1 -> Out1/1

== system blockdiagram/Subsystem1 ==
  In1 : Inport
  If Action Subsystem1 : Subsystem  TreatAsAtomicUnit=on
  If Action Subsystem3 : Subsystem  TreatAsAtomicUnit=on
  If2 : If  IfExpression=u1 <ep
  Merge2 : Merge
  Out1 : Outport
  wires:
  In1/1 -> If Action Subsystem1/1(In1), If Action Subsystem3/1(In1), If2/1
  If2/1 -> If Action Subsystem3/Action
  If2/2 -> If Action Subsystem1/Action
  If Action Subsystem1/1(Out1) -> Merge2/2
  Merge2/1 -> Out1/1
  If Action Subsystem3/1(Out1) -> Merge2/1

== system blockdiagram/Subsystem2 ==
  In1 : Inport
  If Action Subsystem1 : Subsystem  TreatAsAtomicUnit=on
  If Action Subsystem3 : Subsystem  TreatAsAtomicUnit=on
  If2 : If  IfExpression=u1 <ep
  Merge2 : Merge
  Out1 : Outport
  wires:
  In1/1 -> If Action Subsystem1/1(In1), If Action Subsystem3/1(In1), If2/1
  If2/1 -> If Action Subsystem3/Action
  If2/2 -> If Action Subsystem1/Action
  If Action Subsystem1/1(Out1) -> Merge2/2
  Merge2/1 -> Out1/1
  If Action Subsystem3/1(Out1) -> Merge2/1

== system blockdiagram/Subsystem3 ==
  In1 : Inport
  If Action Subsystem1 : Subsystem  TreatAsAtomicUnit=on
  If Action Subsystem3 : Subsystem  TreatAsAtomicUnit=on
  If2 : If  IfExpression=u1 <-ep
  Merge2 : Merge
  Out1 : Outport
  wires:
  In1/1 -> If Action Subsystem1/1(In1), If Action Subsystem3/1(In1), If2/1
  If2/1 -> If Action Subsystem3/Action
  If2/2 -> If Action Subsystem1/Action
  If Action Subsystem1/1(Out1) -> Merge2/2
  Merge2/1 -> Out1/1
  If Action Subsystem3/1(Out1) -> Merge2/1

== system blockdiagram/Subsystem4 ==
  In1 : Inport
  If Action Subsystem1 : Subsystem  TreatAsAtomicUnit=on
  If Action Subsystem3 : Subsystem  TreatAsAtomicUnit=on
  If2 : If  IfExpression=u1 >-ep
  Merge2 : Merge
  Out1 : Outport
  wires:
  In1/1 -> If Action Subsystem1/1(In1), If Action Subsystem3/1(In1), If2/1
  If2/1 -> If Action Subsystem3/Action
  If2/2 -> If Action Subsystem1/Action
  If Action Subsystem1/1(Out1) -> Merge2/2
  Merge2/1 -> Out1/1
  If Action Subsystem3/1(Out1) -> Merge2/1

== system blockdiagram/Subsystem5 ==
  In1 : Inport
  Derivative1 : Derivative
  If Action Subsystem1 : Subsystem  TreatAsAtomicUnit=on
  If Action Subsystem3 : Subsystem  TreatAsAtomicUnit=on
  If2 : If  IfExpression=u1 < 0
  Merge2 : Merge
  Out1 : Outport
  wires:
  Derivative1/1 -> If2/1
  If2/2 -> If Action Subsystem1/Action
  If Action Subsystem1/1(Out1) -> Merge2/2
  If Action Subsystem3/1(Out2) -> Merge2/1
  If2/1 -> If Action Subsystem3/Action
  In1/1 -> If Action Subsystem3/1(In2), If Action Subsystem1/1(In1), Derivative1/1
  Merge2/1 -> Out1/1

== system blockdiagram/Subsystem6 ==
  In1 : Inport
  Derivative1 : Derivative
  If Action Subsystem1 : Subsystem  TreatAsAtomicUnit=on
  If Action Subsystem3 : Subsystem  TreatAsAtomicUnit=on
  If2 : If  IfExpression=u1 < 0
  Merge2 : Merge
  Out1 : Outport
  wires:
  Derivative1/1 -> If2/1
  If2/2 -> If Action Subsystem1/Action
  If Action Subsystem1/1(Out1) -> Merge2/2
  If Action Subsystem3/1(Out2) -> Merge2/1
  If2/1 -> If Action Subsystem3/Action
  In1/1 -> If Action Subsystem3/1(In2), If Action Subsystem1/1(In1), Derivative1/1
  Merge2/1 -> Out1/1

== system blockdiagram/Subsystem7 ==
  In1 : Inport
  Derivative1 : Derivative
  If Action Subsystem1 : Subsystem  TreatAsAtomicUnit=on
  If Action Subsystem3 : Subsystem  TreatAsAtomicUnit=on
  If2 : If  IfExpression=u1 < 0
  Merge2 : Merge
  Out1 : Outport
  wires:
  Derivative1/1 -> If2/1
  If2/2 -> If Action Subsystem1/Action
  If Action Subsystem1/1(Out1) -> Merge2/2
  If Action Subsystem3/1(Out2) -> Merge2/1
  If2/1 -> If Action Subsystem3/Action
  In1/1 -> If Action Subsystem3/1(In2), If Action Subsystem1/1(In1), Derivative1/1
  Merge2/1 -> Out1/1

== system blockdiagram/Subsystem8 ==
  In1 : Inport
  Derivative1 : Derivative
  If Action Subsystem1 : Subsystem  TreatAsAtomicUnit=on
  If Action Subsystem3 : Subsystem  TreatAsAtomicUnit=on
  If2 : If  IfExpression=u1 < 0
  Merge2 : Merge
  Out1 : Outport
  wires:
  Derivative1/1 -> If2/1
  If2/2 -> If Action Subsystem1/Action
  If Action Subsystem1/1(Out1) -> Merge2/2
  If Action Subsystem3/1(Out2) -> Merge2/1
  If2/1 -> If Action Subsystem3/Action
  In1/1 -> If Action Subsystem3/1(In2), If Action Subsystem1/1(In1), Derivative1/1
  Merge2/1 -> Out1/1

== system blockdiagram/wm reference ==
  Demux : Demux  Tag=STV Demux  Outputs=1
      settings: DisplayOption=none
  FromWs : FromWorkspace  Tag=STV FromWs  VariableName=tuvar
      SigBuilderData=|
      | common.afterFinalStr = 'Extrapolate'
      | common.sampleTime = 0
      | dataSet.timeRange = [0 20]
      | dataSet.name = 'Group 1'
      | sbobj.Groups.Name = 'Group 1'
      | sbobj.Groups.Signals.Name = 'Signal 1'
      | sbobj.Groups.Signals.XData = [0 3 3 7 7 20]
      | sbobj.Groups.Signals.YData = [20 20 40 40 -20 -20]
      | sbobj.Groups.TimeRange = [0 20]
  Signal 1 : Outport  Tag=STV Outport
  wires:
  Demux/1 -> Signal 1/1
  FromWs/1 -> Demux/1

== system blockdiagram/wm reference1 ==
  Demux : Demux  Tag=STV Demux  Outputs=1
      settings: DisplayOption=none
  FromWs : FromWorkspace  Tag=STV FromWs  VariableName=tuvar
      SigBuilderData=|
      | common.afterFinalStr = 'Extrapolate'
      | common.sampleTime = 0
      | dataSet.timeRange = [0 20]
      | dataSet.name = 'Group 1'
      | sbobj.Groups.Name = 'Group 1'
      | sbobj.Groups.Signals.Name = 'Signal 1'
      | sbobj.Groups.Signals.XData = [0 4 4 9 9 20]
      | sbobj.Groups.Signals.YData = [20 20 40 40 -20 -20]
      | sbobj.Groups.TimeRange = [0 20]
  Signal 1 : Outport  Tag=STV Outport
  wires:
  Demux/1 -> Signal 1/1
  FromWs/1 -> Demux/1

== system blockdiagram/wm reference2 ==
  Demux : Demux  Tag=STV Demux  Outputs=1
      settings: DisplayOption=none
  FromWs : FromWorkspace  Tag=STV FromWs  VariableName=tuvar
      SigBuilderData=|
      | common.afterFinalStr = 'Extrapolate'
      | common.sampleTime = 0
      | dataSet.timeRange = [0 20]
      | dataSet.name = 'Group 1'
      | sbobj.Groups.Name = 'Group 1'
      | sbobj.Groups.Signals.Name = 'Signal 1'
      | sbobj.Groups.Signals.XData = [0 3 3 7 7 20]
      | sbobj.Groups.Signals.YData = [20 20 40 40 -20 -20]
      | sbobj.Groups.TimeRange = [0 20]
  Signal 1 : Outport  Tag=STV Outport
  wires:
  Demux/1 -> Signal 1/1
  FromWs/1 -> Demux/1

== system blockdiagram/wm reference3 ==
  Demux : Demux  Tag=STV Demux  Outputs=1
      settings: DisplayOption=none
  FromWs : FromWorkspace  Tag=STV FromWs  VariableName=tuvar
      SigBuilderData=|
      | common.afterFinalStr = 'Extrapolate'
      | common.sampleTime = 0
      | dataSet.timeRange = [0 20]
      | dataSet.name = 'Group 1'
      | sbobj.Groups.Name = 'Group 1'
      | sbobj.Groups.Signals.Name = 'Signal 1'
      | sbobj.Groups.Signals.XData = [0 1.25 1.25 20]
      | sbobj.Groups.Signals.YData = [-21.8 -21.8 0 0]
      | sbobj.Groups.TimeRange = [0 20]
  Signal 1 : Outport  Tag=STV Outport
  wires:
  FromWs/1 -> Demux/1
  Demux/1 -> Signal 1/1

== system blockdiagram/wm reference4 ==
  Demux : Demux  Tag=STV Demux  Outputs=1
      settings: DisplayOption=none
  FromWs : FromWorkspace  Tag=STV FromWs  VariableName=tuvar
      SigBuilderData=|
      | common.afterFinalStr = 'Extrapolate'
      | common.sampleTime = 0
      | dataSet.timeRange = [0 20]
      | dataSet.name = 'Group 1'
      | sbobj.Groups.Name = 'Group 1'
      | sbobj.Groups.Signals.Name = 'Signal 1'
      | sbobj.Groups.Signals.XData = [0 3.2 3.2 9 9 20]
      | sbobj.Groups.Signals.YData = [20 20 40 40 -20 -20]
      | sbobj.Groups.TimeRange = [0 20]
  Signal 1 : Outport  Tag=STV Outport
  wires:
  Demux/1 -> Signal 1/1
  FromWs/1 -> Demux/1

== system blockdiagram/wm reference5 ==
  Demux : Demux  Tag=STV Demux  Outputs=1
      settings: DisplayOption=none
  FromWs : FromWorkspace  Tag=STV FromWs  VariableName=tuvar
      SigBuilderData=|
      | common.afterFinalStr = 'Extrapolate'
      | common.sampleTime = 0
      | dataSet.timeRange = [0 20]
      | dataSet.name = 'Group 1'
      | sbobj.Groups.Name = 'Group 1'
      | sbobj.Groups.Signals.Name = 'Signal 1'
      | sbobj.Groups.Signals.XData = [0 1.55 1.55 20]
      | sbobj.Groups.Signals.YData = [-34.4 -34.4 0 0]
      | sbobj.Groups.TimeRange = [0 20]
  Signal 1 : Outport  Tag=STV Outport
  wires:
  FromWs/1 -> Demux/1
  Demux/1 -> Signal 1/1

== system blockdiagram/wm reference6 ==
  Demux : Demux  Tag=STV Demux  Outputs=1
      settings: DisplayOption=none
  FromWs : FromWorkspace  Tag=STV FromWs  VariableName=tuvar
      SigBuilderData=|
      | common.afterFinalStr = 'Extrapolate'
      | common.sampleTime = 0
      | dataSet.timeRange = [0 20]
      | dataSet.name = 'Group 1'
      | sbobj.Groups.Name = 'Group 1'
      | sbobj.Groups.Signals.Name = 'Signal 1'
      | sbobj.Groups.Signals.XData = [0 3 3 7 7 20]
      | sbobj.Groups.Signals.YData = [20 20 40 40 -20 -20]
      | sbobj.Groups.TimeRange = [0 20]
  Signal 1 : Outport  Tag=STV Outport
  wires:
  Demux/1 -> Signal 1/1
  FromWs/1 -> Demux/1

== system blockdiagram/wm reference7 ==
  Demux : Demux  Tag=STV Demux  Outputs=1
      settings: DisplayOption=none
  FromWs : FromWorkspace  Tag=STV FromWs  VariableName=tuvar
      SigBuilderData=|
      | common.afterFinalStr = 'Extrapolate'
      | common.sampleTime = 0
      | dataSet.timeRange = [0 20]
      | dataSet.name = 'Group 1'
      | sbobj.Groups.Name = 'Group 1'
      | sbobj.Groups.Signals.Name = 'Signal 1'
      | sbobj.Groups.Signals.XData = [0 3 3 7 7 20]
      | sbobj.Groups.Signals.YData = [20 20 40 40 -20 -20]
      | sbobj.Groups.TimeRange = [0 20]
  Signal 1 : Outport  Tag=STV Outport
  wires:
  Demux/1 -> Signal 1/1
  FromWs/1 -> Demux/1

== system blockdiagram/If Action Subsystem1/If Action Subsystem2 ==
  In1 : Inport
  Action Port : ActionPort  ActionPortLabel=else
  Constant14 : Constant  Value=2*pi
  Mod13 : Math  Operator=mod  SaturateOnIntegerOverflow=on
  Out1 : Outport
  wires:
  In1/1 -> Mod13/1
  Constant14/1 -> Mod13/2
  Mod13/1 -> Out1/1

== system blockdiagram/If Action Subsystem1/If Action Subsystem4 ==
  In1 : Inport
  Action Port : ActionPort  InitializeStates=reset  ActionPortLabel=if(u1 <ep)
  Out1 : Outport
  wires:
  In1/1 -> Out1/1

== system blockdiagram/If Action Subsystem2/If Action Subsystem2 ==
  In1 : Inport
  Action Port : ActionPort  ActionPortLabel=else
  Constant14 : Constant  Value=2*pi
  Mod13 : Math  Operator=mod  SaturateOnIntegerOverflow=on
  Out1 : Outport
  wires:
  In1/1 -> Mod13/1
  Constant14/1 -> Mod13/2
  Mod13/1 -> Out1/1

== system blockdiagram/If Action Subsystem2/If Action Subsystem4 ==
  In1 : Inport
  Action Port : ActionPort  InitializeStates=reset  ActionPortLabel=if(u1 <ep)
  Out1 : Outport
  wires:
  In1/1 -> Out1/1

== system blockdiagram/If Action Subsystem3/If Action Subsystem1 ==
  In1 : Inport
  Action Port : ActionPort  ActionPortLabel=else
  Constant14 : Constant  Value=-2*pi
  Mod13 : Math  Operator=mod  SaturateOnIntegerOverflow=on
  Out1 : Outport
  wires:
  In1/1 -> Mod13/1
  Constant14/1 -> Mod13/2
  Mod13/1 -> Out1/1
